simulink model "homework4"  (R2024a)
settings: Solver=FixedStepAuto  StartTime=0.0  StopTime=10.0  RelTol=1e-3
libraries: robotlib x5
settings Model: Creator=katiegildersleeve  LastModifiedBy=katiegildersleeve
settings OptimizationCC: EnhancedBackFolding=on  PassReuseOutputArgsAs=Individual arguments  ZeroExternalMemoryAtStartup=off  ZeroInternalMemoryAtStartup=off  MaxStackSize=64  OptimizeBlockOrder=speed  DifferentSizesBufferReuse=on  OptimizationCustomize=off  EfficientTunableParamExpr=on
settings DebuggingCC: ParameterTunabilityLossMsg=error
settings HardwareCC: ProdBitPerPointer=32  ProdBitPerSizeT=32  ProdBitPerPtrDiffT=32  ProdLargestAtomicFloat=None  ProdIntDivRoundTo=Undefined  ProdEndianess=Unspecified  ProdWordSize=32  ProdHWDeviceType=Generic->Unspecified (assume 32-bit Generic)  UseEmbeddedCoderFeatures=off
settings SFSimCC: MATLABDynamicMemAlloc=off
settings RTWCC: Description=Embedded Coder  SystemTargetFile=ert.tlc  HardwareBoard=Robot Operating System (ROS)  TLCOptions="-aInlineSetEventsForThisBaseRateFcn=TLC_FALSE -aSuppressMultiTaskScheduler=TLC_FALSE  -aRateBasedStepFcn=0"  TemplateMakefile=ert_default_tmf  Toolchain=Catkin  TargetLang=C++
settings CodeAppCC: ForceParamTrailComments=on  IgnoreCustomStorageClasses=off  OperatorAnnotations=on  SimulinkDataObjDesc=on  SFDataObjDesc=on  InsertBlockDesc=on
settings ERTTargetCC: SupportNonInlinedSFcns=on

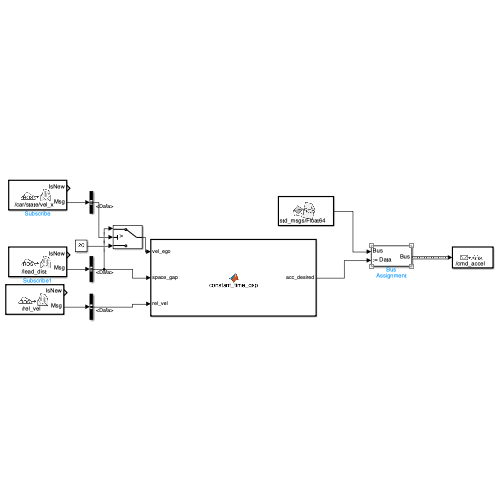
[thumbnail: Simulink's stored preview of the top-level diagram]
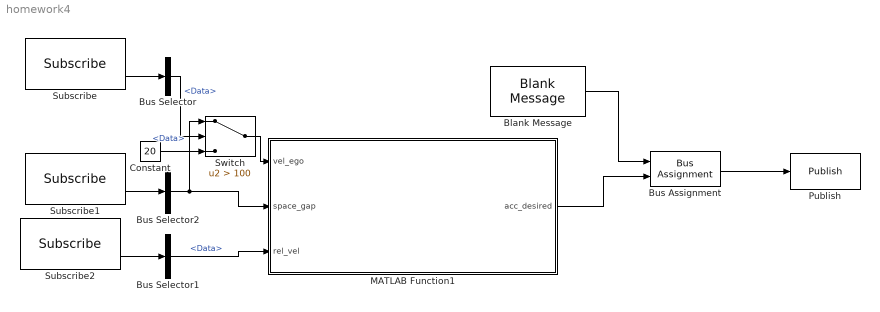
== system homework4 ==
  Blank Message : robotlib/Blank Message  messageClass=Message  entityType=std_msgs/Float64  messageType=std_msgs/Float64  SampleTime=inf  legacyBusStruct=off
  Bus Assignment : BusAssignment  AssignedSignals=Data
  Bus Selector : BusSelector  OutputSignals=Data
  Bus Selector1 : BusSelector  OutputSignals=Data
  Bus Selector2 : BusSelector  OutputSignals=Data
  Constant : Constant  Value=20
  MATLAB Function1 : MATLAB Function  TreatAsAtomicUnit=on
  Publish : robotlib/Publish  topicSource=Specify your own  topic=/cmd_accel  messageType=std_msgs/Float64  legacyBusStruct=off  messageQueueLength=1
  Subscribe : robotlib/Subscribe  topicSource=Specify your own  topic=/car/state/vel_x  messageType=std_msgs/Float64  SampleTime=-1  legacyBusStruct=off  messageQueueLength=1
  Subscribe1 : robotlib/Subscribe  topicSource=Specify your own  topic=/lead_dist  messageType=std_msgs/Float64  SampleTime=-1  legacyBusStruct=off  messageQueueLength=1
  Subscribe2 : robotlib/Subscribe  topicSource=Specify your own  topic=/rel_vel  messageType=std_msgs/Float64  SampleTime=-1  legacyBusStruct=off  messageQueueLength=1
  Switch : Switch  Criteria=u2 > Threshold  Threshold=100  SaturateOnIntegerOverflow=off  InputSameDT=off
  wires:
  Bus Selector1/1 -> MATLAB Function1/3(rel_vel)  "<Data>"
  Bus Selector2/1 -> Switch/1, MATLAB Function1/2(space_gap)  "<Data>"
  Bus Assignment/1 -> Publish/1
  MATLAB Function1/1(acc_desired) -> Bus Assignment/2
  Switch/1 -> MATLAB Function1/1(vel_ego)
  Constant/1 -> Switch/3
  Bus Selector/1 -> Switch/2  "<Data>"
  Subscribe/2 -> Bus Selector/1
  Subscribe1/2 -> Bus Selector2/1
  Subscribe2/2 -> Bus Selector1/1
  Blank Message/1 -> Bus Assignment/1

== matlab function homework4/MATLAB Function1 ==
  data: vel_ego input; space_gap input; acc_desired output; rel_vel input
function acc_desired  = constant_time_gap(vel_ego, space_gap, rel_vel)

alpha = 0.25;
tau_desired = 2.0;

if space_gap < 0
    acc_desired = 0;
else

    if vel_ego > -0.01 && vel_ego < 0.01 % to avoid dividing by zero
        vel_ego = 0.01;
    end
    acc_desired = alpha*(((space_gap)/vel_ego) - tau_desired) + rel_vel;
end
